simulink model "aurora_cpu_ch0_ver2_rtxsg"  (R2019b)
settings: Solver=ode45  StartTime=0.0  StopTime=1/6000  RelTol=1e-3  EnableMultiTasking=on
PreLoadFcn:
  | period=5e-9;
InitFcn:
  | period=5e-9;
undefined symbols (not defined in the file): DUALSFP, EX, opGetFPGAPeriod, VC707_2
libraries: xbsIndex_r4 x170, rtxsg_tools x22, rtxsg_communication x3, rtxsg_common x3, HighSpeedCommIO_lib x2, rtxsg_serdes_lib x2, vc707_lib x1
(part 4 of 4)

== system aurora_cpu_ch0_ver2_rtxsg/SOF_detector ==
  ready : Inport
  last : Inport  Port=2
  Inverter4 : xbsIndex_r4/Inverter  en=off  latency=0  dbl_ovrd=off  block_type=inv
  Logical1 : xbsIndex_r4/Logical  logical_function=OR  inputs=2  en=off  latency=0  precision=Full  arith_type=Unsigned  n_bits=16  bin_pt=0  align_bp=on  dbl_ovrd=off  block_type=logical
  Logical5 : xbsIndex_r4/Logical  logical_function=AND  inputs=2  en=off  latency=0  precision=Full  arith_type=Unsigned  n_bits=16  bin_pt=0  align_bp=on  dbl_ovrd=off  block_type=logical
  Register3 : xbsIndex_r4/Register  init=0  rst=on  en=off  dbl_ovrd=off  block_type=register
  startofframe : Outport
  wires:
  Register3/1 -> Logical1/1, Inverter4/1
  ready/1 -> Logical1/2, Logical5/2
  Inverter4/1 -> Logical5/1
  Logical1/1 -> Register3/1
  Logical5/1 -> startofframe/1
  last/1 -> Register3/2

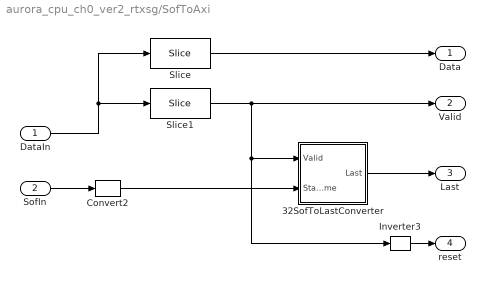
== system aurora_cpu_ch0_ver2_rtxsg/SofToAxi ==
  DataIn : Inport
  SofIn : Inport  Port=2
  32SofToLastConverter : Subsystem
  Convert2 : xbsIndex_r4/Convert  gui_display_data_type=Boolean  arith_type=Boolean  n_bits=16  bin_pt=14  float_type=Single  exp_bits=8  fraction_bits=24  quantization=Truncate  overflow=Wrap  en=off  latency=0  pipeline=off  dbl_ovrd=off  block_type=convert
  Inverter3 : xbsIndex_r4/Inverter  en=off  latency=0  dbl_ovrd=off  block_type=inv
  Slice : xbsIndex_r4/Slice  nbits=32  boolean_output=off  mode=Upper Bit Location + Width  bit1=31  base1=LSB of Input  bit0=0  base0=LSB of Input  dbl_ovrd=off  block_type=slice
  Slice1 : xbsIndex_r4/Slice  nbits=1  boolean_output=on  mode=Upper Bit Location + Width  bit1=32  base1=LSB of Input  bit0=32  base0=LSB of Input  dbl_ovrd=off  block_type=slice
  Data : Outport
  Valid : Outport  Port=2
  Last : Outport  Port=3
  reset : Outport  Port=4
  wires:
  DataIn/1 -> Slice/1, Slice1/1
  32SofToLastConverter/1(Last) -> Last/1
  Convert2/1 -> 32SofToLastConverter/2(StartOfFrame)
  Slice1/1 -> Valid/1, Inverter3/1, 32SofToLastConverter/1(Valid)
  Slice/1 -> Data/1
  SofIn/1 -> Convert2/1
  Inverter3/1 -> reset/1

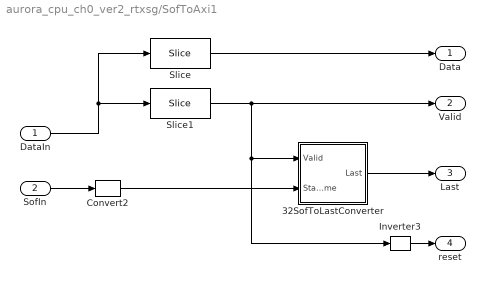
== system aurora_cpu_ch0_ver2_rtxsg/SofToAxi1 ==
  DataIn : Inport
  SofIn : Inport  Port=2
  32SofToLastConverter : Subsystem
  Convert2 : xbsIndex_r4/Convert  gui_display_data_type=Boolean  arith_type=Boolean  n_bits=16  bin_pt=14  float_type=Single  exp_bits=8  fraction_bits=24  quantization=Truncate  overflow=Wrap  en=off  latency=0  pipeline=off  dbl_ovrd=off  block_type=convert
  Inverter3 : xbsIndex_r4/Inverter  en=off  latency=0  dbl_ovrd=off  block_type=inv
  Slice : xbsIndex_r4/Slice  nbits=32  boolean_output=off  mode=Upper Bit Location + Width  bit1=31  base1=LSB of Input  bit0=0  base0=LSB of Input  dbl_ovrd=off  block_type=slice
  Slice1 : xbsIndex_r4/Slice  nbits=1  boolean_output=on  mode=Upper Bit Location + Width  bit1=32  base1=LSB of Input  bit0=32  base0=LSB of Input  dbl_ovrd=off  block_type=slice
  Data : Outport
  Valid : Outport  Port=2
  Last : Outport  Port=3
  reset : Outport  Port=4
  wires:
  DataIn/1 -> Slice/1, Slice1/1
  32SofToLastConverter/1(Last) -> Last/1
  Convert2/1 -> 32SofToLastConverter/2(StartOfFrame)
  Slice1/1 -> Valid/1, Inverter3/1, 32SofToLastConverter/1(Valid)
  Slice/1 -> Data/1
  SofIn/1 -> Convert2/1
  Inverter3/1 -> reset/1

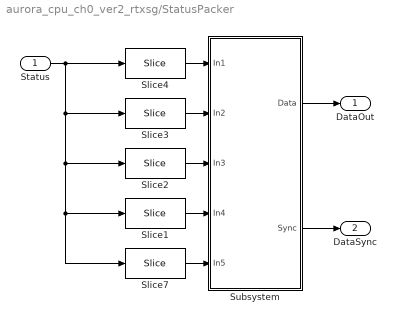
== system aurora_cpu_ch0_ver2_rtxsg/StatusPacker ==
  Status : Inport
  Slice1 : xbsIndex_r4/Slice  nbits=16  boolean_output=off  mode=Lower Bit Location + Width  bit1=0  base1=MSB of Input  bit0=80  base0=LSB of Input  dbl_ovrd=off  block_type=slice
  Slice2 : xbsIndex_r4/Slice  nbits=32  boolean_output=off  mode=Lower Bit Location + Width  bit1=0  base1=MSB of Input  bit0=48  base0=LSB of Input  dbl_ovrd=off  block_type=slice
  Slice3 : xbsIndex_r4/Slice  nbits=16  boolean_output=off  mode=Lower Bit Location + Width  bit1=0  base1=MSB of Input  bit0=32  base0=LSB of Input  dbl_ovrd=off  block_type=slice
  Slice4 : xbsIndex_r4/Slice  nbits=32  boolean_output=off  mode=Lower Bit Location + Width  bit1=0  base1=MSB of Input  bit0=0  base0=LSB of Input  dbl_ovrd=off  block_type=slice
  Slice7 : xbsIndex_r4/Slice  nbits=6  boolean_output=off  mode=Lower Bit Location + Width  bit1=0  base1=MSB of Input  bit0=96  base0=LSB of Input  dbl_ovrd=off  block_type=slice
  Subsystem : Subsystem
  DataOut : Outport
  DataSync : Outport  Port=2
  wires:
  Subsystem/1(Data) -> DataOut/1
  Subsystem/2(Sync) -> DataSync/1
  Status/1 -> Slice4/1, Slice3/1, Slice2/1, Slice1/1, Slice7/1
  Slice4/1 -> Subsystem/1(In1)
  Slice3/1 -> Subsystem/2(In2)
  Slice2/1 -> Subsystem/3(In3)
  Slice1/1 -> Subsystem/4(In4)
  Slice7/1 -> Subsystem/5(In5)

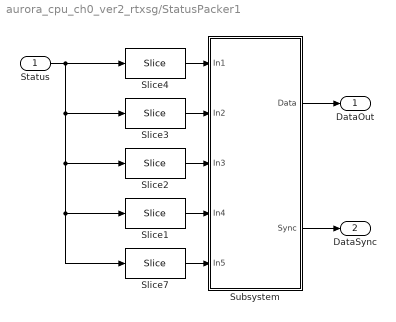
== system aurora_cpu_ch0_ver2_rtxsg/StatusPacker1 ==
  Status : Inport
  Slice1 : xbsIndex_r4/Slice  nbits=16  boolean_output=off  mode=Lower Bit Location + Width  bit1=0  base1=MSB of Input  bit0=80  base0=LSB of Input  dbl_ovrd=off  block_type=slice
  Slice2 : xbsIndex_r4/Slice  nbits=32  boolean_output=off  mode=Lower Bit Location + Width  bit1=0  base1=MSB of Input  bit0=48  base0=LSB of Input  dbl_ovrd=off  block_type=slice
  Slice3 : xbsIndex_r4/Slice  nbits=16  boolean_output=off  mode=Lower Bit Location + Width  bit1=0  base1=MSB of Input  bit0=32  base0=LSB of Input  dbl_ovrd=off  block_type=slice
  Slice4 : xbsIndex_r4/Slice  nbits=32  boolean_output=off  mode=Lower Bit Location + Width  bit1=0  base1=MSB of Input  bit0=0  base0=LSB of Input  dbl_ovrd=off  block_type=slice
  Slice7 : xbsIndex_r4/Slice  nbits=6  boolean_output=off  mode=Lower Bit Location + Width  bit1=0  base1=MSB of Input  bit0=96  base0=LSB of Input  dbl_ovrd=off  block_type=slice
  Subsystem : Subsystem
  DataOut : Outport
  DataSync : Outport  Port=2
  wires:
  Subsystem/1(Data) -> DataOut/1
  Subsystem/2(Sync) -> DataSync/1
  Status/1 -> Slice4/1, Slice3/1, Slice2/1, Slice1/1, Slice7/1
  Slice4/1 -> Subsystem/1(In1)
  Slice3/1 -> Subsystem/2(In2)
  Slice2/1 -> Subsystem/3(In3)
  Slice1/1 -> Subsystem/4(In4)
  Slice7/1 -> Subsystem/5(In5)

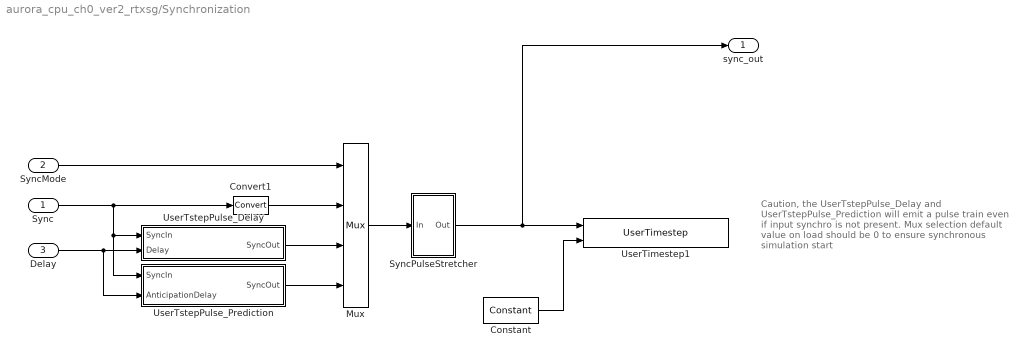
== system aurora_cpu_ch0_ver2_rtxsg/Synchronization ==
  note: Caution, the UserTstepPulse_Delay and
      | UserTstepPulse_Prediction will emit a pulse train
      | even if input synchro is not present. Mux selection
      | default value on load should be 0 to ensure
      | synchronous simulation start
  Sync : Inport
  SyncMode : Inport  Port=2
  Delay : Inport  Port=3
  Constant : xbsIndex_r4/Constant  const=1.0  gui_display_data_type=Fixed-point  arith_type=Unsigned  n_bits=1  bin_pt=0  preci_type=Single  exp_width=8  frac_width=24  explicit_period=on  period=opGetFPGAPeriod(bdroot)  equ=P=C  opselect=C  inp2=PCIN>>17  opr=+  inp1=P  carry=CIN  dbl_ovrd=off  block_type=constant
  Convert1 : xbsIndex_r4/Convert  gui_display_data_type=Boolean  arith_type=Boolean  n_bits=1  bin_pt=0  float_type=Single  exp_bits=8  fraction_bits=24  quantization=Truncate  overflow=Wrap  en=off  latency=0  pipeline=off  dbl_ovrd=off  block_type=convert
  Mux : xbsIndex_r4/Mux  inputs=3  en=off  latency=0  precision=Full  arith_type=Unsigned  n_bits=16  bin_pt=14  quantization=Truncate  overflow=Wrap  dbl_ovrd=off  block_type=mux
  SyncPulseStretcher : Subsystem
  UserTimestep1 : vc707_lib/UserTimestep  SyncSelControl=From Input Port  SamplePeriod=opGetFPGAPeriod(bdroot)
      link override SyncSelCtrl: const=0  gui_display_data_type=Fixed-point  arith_type=Unsigned  n_bits=1  bin_pt=0  preci_type=Single  exp_width=8  frac_width=24  explicit_period=on  period=SamplePeriod  equ=P=C  opselect=C  inp2=PCIN>>17  opr=+  inp1=P  carry=CIN  dbl_ovrd=off
      settings: SourceProductName=RT-XSG
  UserTstepPulse_Delay : Subsystem
  UserTstepPulse_Prediction : Subsystem
  sync_out : Outport
  wires:
  Sync/1 -> UserTstepPulse_Prediction/1(SyncIn), UserTstepPulse_Delay/1(SyncIn), Convert1/1
  SyncMode/1 -> Mux/1
  Delay/1 -> UserTstepPulse_Prediction/2(AnticipationDelay), UserTstepPulse_Delay/2(Delay)
  Convert1/1 -> Mux/2
  UserTstepPulse_Delay/1(SyncOut) -> Mux/3
  UserTstepPulse_Prediction/1(SyncOut) -> Mux/4
  SyncPulseStretcher/1(Out) -> sync_out/1, UserTimestep1/1
  Constant/1 -> UserTimestep1/2
  Mux/1 -> SyncPulseStretcher/1(In)

== system aurora_cpu_ch0_ver2_rtxsg/TimeStepSwitch ==
  MasterTimeStep : Inport
  InitTimeStep : Inport  Port=2
  Logical : xbsIndex_r4/Logical  logical_function=OR  inputs=2  en=off  latency=0  precision=Full  arith_type=Unsigned  n_bits=16  bin_pt=0  align_bp=on  dbl_ovrd=off  block_type=logical
  Mux : xbsIndex_r4/Mux  inputs=2  en=off  latency=0  precision=Full  arith_type=Unsigned  n_bits=16  bin_pt=14  quantization=Truncate  overflow=Wrap  dbl_ovrd=off  block_type=mux
  Register : xbsIndex_r4/Register  init=0  rst=off  en=off  dbl_ovrd=off  block_type=register
  TimeStep : Outport
  wires:
  Register/1 -> Logical/1
  MasterTimeStep/1 -> Logical/2, Mux/3
  Logical/1 -> Mux/1, Register/1
  Mux/1 -> TimeStep/1
  InitTimeStep/1 -> Mux/2

== system aurora_cpu_ch0_ver2_rtxsg/TimestepGenerator ==
  Constant3 : xbsIndex_r4/Constant  const=5000  gui_display_data_type=Fixed-point  arith_type=Unsigned  n_bits=32  bin_pt=0  preci_type=Single  exp_width=8  frac_width=24  explicit_period=on  period=opGetFPGAPeriod(bdroot)  equ=P=C  opselect=C  inp2=PCIN>>17  opr=+  inp1=P  carry=CIN  dbl_ovrd=off  block_type=constant
  Counter1 : xbsIndex_r4/Counter  cnt_type=Free Running  cnt_to=50e-6/1e-9  operation=Up  start_count=0  cnt_by_val=1  arith_type=Unsigned  n_bits=32  bin_pt=0  load_pin=off  rst=on  en=off  explicit_period=on  period=opGetFPGAPeriod(bdroot)  use_behavioral_HDL=off  implementation=Fabric  dbl_ovrd=off  block_type=counter
  Relational : xbsIndex_r4/Relational  mode=a=b  op_type=Bool  en=off  latency=0  dbl_ovrd=off  block_type=relational
  TimeStep : Outport
  wires:
  Relational/1 -> TimeStep/1, Counter1/1
  Constant3/1 -> Relational/2
  Counter1/1 -> Relational/1

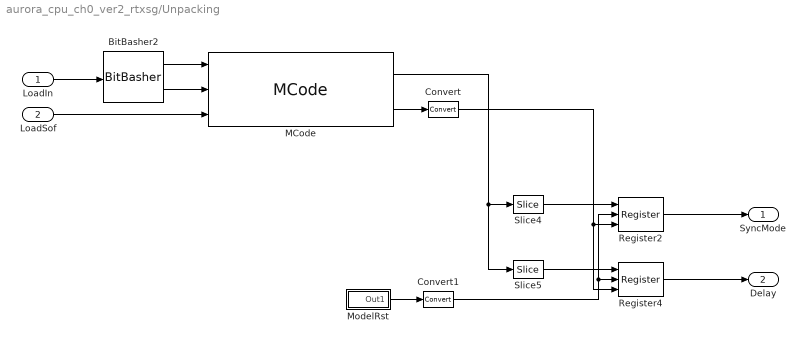
== system aurora_cpu_ch0_ver2_rtxsg/Unpacking ==
  LoadIn : Inport
  LoadSof : Inport  Port=2
  BitBasher2 : xbsIndex_r4/BitBasher  bitexpr=|  display_expr=off  sr_1=1  arith_type1=Unsigned  bin_pt1=0  sr_2=2  arith_type2=Unsigned  bin_pt2=0  sr_3=3  arith_type3=Unsigned  bin_pt3=0  sr_4=4  arith_type4=Unsigned  bin_pt4=0  dbl_ovrd=off  block_type=bitbasher
      | <!DOCTYPE HTML PUBLIC "-//W3C//DTD HTML 4.0//EN" "http://www.w3.org/TR/REC-html40/strict.dtd">
      | <html><head><meta name="qrichtext" content="1" /><style type="text/css">
      | p, li { white-space: pre-wrap; }
      | </style></head><body style=" font-family:'MS Shell Dlg 2'; font-size:8.25pt; font-weight:400; font-style:normal;">
      | <p style=" margin-top:12px; margin-bottom:12px; margin-left:0px; margin-right:0px; -qt-block-indent:0; text-indent:0px;"><span style=" font-family:'MS Shell Dlg'; font-size:8pt;">data={i[31:0]}<br />valid={i[32]}</span></p></body></html>
  Convert : xbsIndex_r4/Convert  gui_display_data_type=Boolean  arith_type=Boolean  n_bits=16  bin_pt=14  float_type=Single  exp_bits=8  fraction_bits=24  quantization=Truncate  overflow=Wrap  en=off  latency=0  pipeline=off  dbl_ovrd=off  block_type=convert
  Convert1 : xbsIndex_r4/Convert  gui_display_data_type=Boolean  arith_type=Boolean  n_bits=16  bin_pt=14  float_type=Single  exp_bits=8  fraction_bits=24  quantization=Truncate  overflow=Wrap  en=off  latency=0  pipeline=off  dbl_ovrd=off  block_type=convert
  MCode : xbsIndex_r4/MCode  mfname=efsUnpackingDesequencerSof  explicit_period=off  period=1  inputsTable={'boundInpExpr'=>['2','','',''],'inputs'=>['NbElements','Output_in','WE','Sof']}  outputsTable={'outputs'=>['Output_cat','OutputUpdated'],'suppressOut'=>['off','off']}  enable_stdout=off  enable_debug=off  suppress_output=on  defparams={'NbElements',2}  hide_port_list={}  dbl_ovrd=off  block_type=mcode
  ModelRst : Subsystem
  Register2 : xbsIndex_r4/Register  init=0  rst=on  en=on  dbl_ovrd=off  block_type=register
  Register4 : xbsIndex_r4/Register  init=0  rst=on  en=on  dbl_ovrd=off  block_type=register
  Slice4 : xbsIndex_r4/Slice  nbits=2  boolean_output=off  mode=Lower Bit Location + Width  bit1=0  base1=MSB of Input  bit0=0  base0=LSB of Input  dbl_ovrd=off  block_type=slice
  Slice5 : xbsIndex_r4/Slice  nbits=22  boolean_output=off  mode=Lower Bit Location + Width  bit1=0  base1=MSB of Input  bit0=2  base0=LSB of Input  dbl_ovrd=off  block_type=slice
  SyncMode : Outport
  Delay : Outport  Port=2
  wires:
  BitBasher2/1 -> MCode/1
  BitBasher2/2 -> MCode/2
  LoadIn/1 -> BitBasher2/1
  LoadSof/1 -> MCode/3
  ModelRst/1(Out1) -> Convert1/1
  MCode/2 -> Convert/1
  MCode/1 -> Slice4/1, Slice5/1
  Register2/1 -> SyncMode/1
  Register4/1 -> Delay/1
  Slice4/1 -> Register2/1
  Slice5/1 -> Register4/1
  Convert/1 -> Register2/3, Register4/3
  Convert1/1 -> Register2/2, Register4/2

== system aurora_cpu_ch0_ver2_rtxsg/SofToAxi/32SofToLastConverter ==
  Valid : Inport
  StartOfFrame : Inport  Port=2
  Constant2 : xbsIndex_r4/Constant  const=31  gui_display_data_type=Fixed-point  arith_type=Signed (2's comp)  n_bits=8  bin_pt=0  preci_type=Single  exp_width=8  frac_width=24  explicit_period=off  period=1  equ=P=C  opselect=C  inp2=PCIN>>17  opr=+  inp1=P  carry=CIN  dbl_ovrd=off  block_type=constant
  Counter : xbsIndex_r4/Counter  cnt_type=Free Running  cnt_to=31  operation=Up  start_count=0  cnt_by_val=1  arith_type=Unsigned  n_bits=8  bin_pt=0  load_pin=off  rst=on  en=on  explicit_period=off  period=1  use_behavioral_HDL=off  implementation=Fabric  dbl_ovrd=off  block_type=counter
  Relational1 : xbsIndex_r4/Relational  mode=a=b  op_type=Bool  en=off  latency=0  dbl_ovrd=off  block_type=relational
  Last : Outport
  wires:
  Counter/1 -> Relational1/2
  Constant2/1 -> Relational1/1
  Valid/1 -> Counter/2
  Relational1/1 -> Last/1
  StartOfFrame/1 -> Counter/1

== system aurora_cpu_ch0_ver2_rtxsg/SofToAxi1/32SofToLastConverter ==
  Valid : Inport
  StartOfFrame : Inport  Port=2
  Constant2 : xbsIndex_r4/Constant  const=31  gui_display_data_type=Fixed-point  arith_type=Signed (2's comp)  n_bits=8  bin_pt=0  preci_type=Single  exp_width=8  frac_width=24  explicit_period=off  period=1  equ=P=C  opselect=C  inp2=PCIN>>17  opr=+  inp1=P  carry=CIN  dbl_ovrd=off  block_type=constant
  Counter : xbsIndex_r4/Counter  cnt_type=Free Running  cnt_to=31  operation=Up  start_count=0  cnt_by_val=1  arith_type=Unsigned  n_bits=8  bin_pt=0  load_pin=off  rst=on  en=on  explicit_period=off  period=1  use_behavioral_HDL=off  implementation=Fabric  dbl_ovrd=off  block_type=counter
  Relational1 : xbsIndex_r4/Relational  mode=a=b  op_type=Bool  en=off  latency=0  dbl_ovrd=off  block_type=relational
  Last : Outport
  wires:
  Counter/1 -> Relational1/2
  Constant2/1 -> Relational1/1
  Valid/1 -> Counter/2
  Relational1/1 -> Last/1
  StartOfFrame/1 -> Counter/1

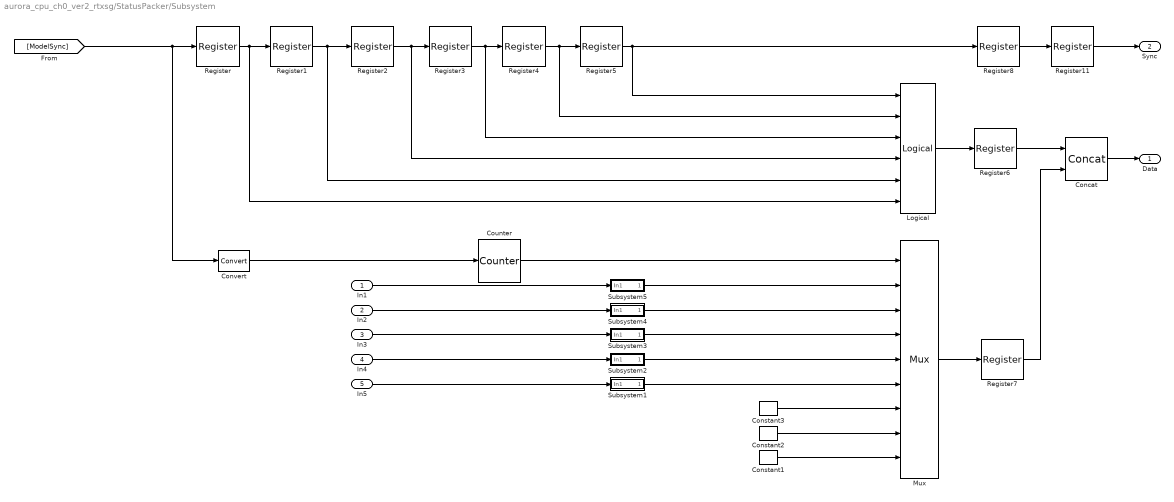
== system aurora_cpu_ch0_ver2_rtxsg/StatusPacker/Subsystem ==
  In1 : Inport
  In2 : Inport  Port=2
  In3 : Inport  Port=3
  In4 : Inport  Port=4
  In5 : Inport  Port=5
  Concat : xbsIndex_r4/Concat  num_inputs=2  dbl_ovrd=off  block_type=concat
  Constant1 : xbsIndex_r4/Constant  const=0  gui_display_data_type=Fixed-point  arith_type=Unsigned  n_bits=32  bin_pt=0  preci_type=Single  exp_width=8  frac_width=24  explicit_period=on  period=opGetFPGAPeriod(bdroot)  equ=P=C  opselect=C  inp2=PCIN>>17  opr=+  inp1=P  carry=CIN  dbl_ovrd=off  block_type=constant
  Constant2 : xbsIndex_r4/Constant  const=0  gui_display_data_type=Fixed-point  arith_type=Unsigned  n_bits=32  bin_pt=0  preci_type=Single  exp_width=8  frac_width=24  explicit_period=on  period=opGetFPGAPeriod(bdroot)  equ=P=C  opselect=C  inp2=PCIN>>17  opr=+  inp1=P  carry=CIN  dbl_ovrd=off  block_type=constant
  Constant3 : xbsIndex_r4/Constant  const=0  gui_display_data_type=Fixed-point  arith_type=Unsigned  n_bits=32  bin_pt=0  preci_type=Single  exp_width=8  frac_width=24  explicit_period=on  period=opGetFPGAPeriod(bdroot)  equ=P=C  opselect=C  inp2=PCIN>>17  opr=+  inp1=P  carry=CIN  dbl_ovrd=off  block_type=constant
  Convert : xbsIndex_r4/Convert  gui_display_data_type=Boolean  arith_type=Boolean  n_bits=16  bin_pt=14  float_type=Single  exp_bits=8  fraction_bits=24  quantization=Truncate  overflow=Wrap  en=off  latency=0  pipeline=off  dbl_ovrd=off  block_type=convert
  Counter : xbsIndex_r4/Counter  cnt_type=Free Running  cnt_to=Inf  operation=Up  start_count=0  cnt_by_val=1  arith_type=Unsigned  n_bits=3  bin_pt=0  load_pin=off  rst=on  en=off  explicit_period=on  period=opGetFPGAPeriod(bdroot)  use_behavioral_HDL=off  implementation=Fabric  dbl_ovrd=off  block_type=counter
  Logical : xbsIndex_r4/Logical  logical_function=OR  inputs=6  en=off  latency=0  precision=Full  arith_type=Unsigned  n_bits=16  bin_pt=0  align_bp=on  dbl_ovrd=off  block_type=logical
  Mux : xbsIndex_r4/Mux  inputs=8  en=off  latency=0  precision=Full  arith_type=Unsigned  n_bits=16  bin_pt=14  quantization=Truncate  overflow=Wrap  dbl_ovrd=off  block_type=mux
  Register{,1..8,11} (10 alike) : xbsIndex_r4/Register  init=0  rst=off  en=off  dbl_ovrd=off  block_type=register
  Subsystem1 : Subsystem
  Subsystem2 : Subsystem
  Subsystem3 : Subsystem
  Subsystem4 : Subsystem
  Subsystem5 : Subsystem
  Data : Outport
  Sync : Outport  Port=2
  wires:
  Convert/1 -> Counter/1
  Concat/1 -> Data/1
  Register7/1 -> Concat/2
  Register6/1 -> Concat/1
  Counter/1 -> Mux/1
  In5/1 -> Subsystem1/1(In1)
  In4/1 -> Subsystem2/1(In1)
  In3/1 -> Subsystem3/1(In1)
  In2/1 -> Subsystem4/1(In1)
  In1/1 -> Subsystem5/1(In1)
  Mux/1 -> Register7/1
  Logical/1 -> Register6/1
  [ModelSync] -> Convert/1, Register/1
  Register5/1 -> Register8/1, Logical/1
  Register4/1 -> Register5/1, Logical/2
  Register3/1 -> Register4/1, Logical/3
  Register2/1 -> Register3/1, Logical/4
  Register1/1 -> Register2/1, Logical/5
  Register/1 -> Register1/1, Logical/6
  Register8/1 -> Register11/1
  Register11/1 -> Sync/1
  Constant2/1 -> Mux/8
  Constant1/1 -> Mux/9
  Subsystem1/1(Out1) -> Mux/6
  Subsystem2/1(Out1) -> Mux/5
  Subsystem3/1(Out1) -> Mux/4
  Subsystem4/1(Out1) -> Mux/3
  Subsystem5/1(Out1) -> Mux/2
  Constant3/1 -> Mux/7

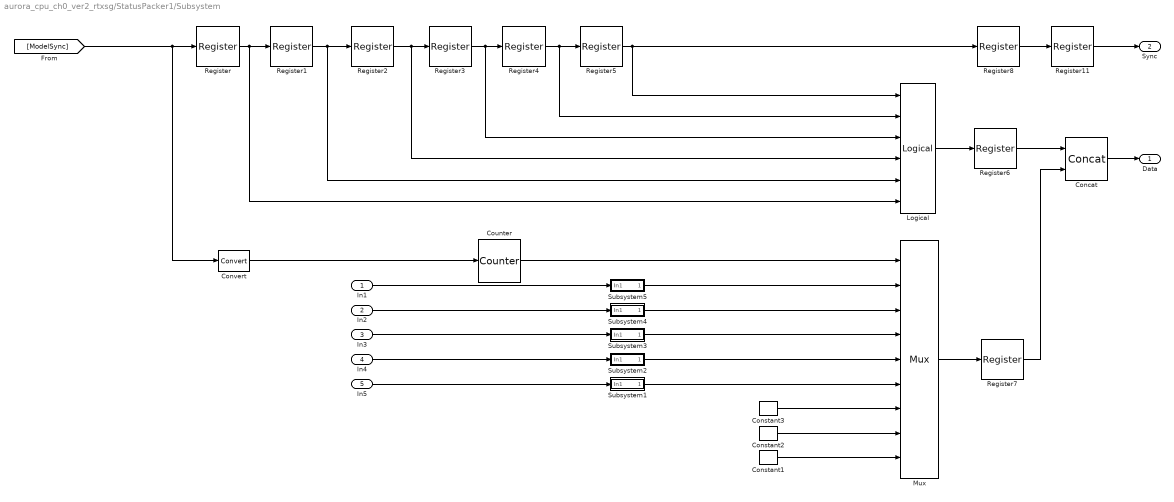
== system aurora_cpu_ch0_ver2_rtxsg/StatusPacker1/Subsystem ==
  In1 : Inport
  In2 : Inport  Port=2
  In3 : Inport  Port=3
  In4 : Inport  Port=4
  In5 : Inport  Port=5
  Concat : xbsIndex_r4/Concat  num_inputs=2  dbl_ovrd=off  block_type=concat
  Constant1 : xbsIndex_r4/Constant  const=0  gui_display_data_type=Fixed-point  arith_type=Unsigned  n_bits=32  bin_pt=0  preci_type=Single  exp_width=8  frac_width=24  explicit_period=on  period=opGetFPGAPeriod(bdroot)  equ=P=C  opselect=C  inp2=PCIN>>17  opr=+  inp1=P  carry=CIN  dbl_ovrd=off  block_type=constant
  Constant2 : xbsIndex_r4/Constant  const=0  gui_display_data_type=Fixed-point  arith_type=Unsigned  n_bits=32  bin_pt=0  preci_type=Single  exp_width=8  frac_width=24  explicit_period=on  period=opGetFPGAPeriod(bdroot)  equ=P=C  opselect=C  inp2=PCIN>>17  opr=+  inp1=P  carry=CIN  dbl_ovrd=off  block_type=constant
  Constant3 : xbsIndex_r4/Constant  const=0  gui_display_data_type=Fixed-point  arith_type=Unsigned  n_bits=32  bin_pt=0  preci_type=Single  exp_width=8  frac_width=24  explicit_period=on  period=opGetFPGAPeriod(bdroot)  equ=P=C  opselect=C  inp2=PCIN>>17  opr=+  inp1=P  carry=CIN  dbl_ovrd=off  block_type=constant
  Convert : xbsIndex_r4/Convert  gui_display_data_type=Boolean  arith_type=Boolean  n_bits=16  bin_pt=14  float_type=Single  exp_bits=8  fraction_bits=24  quantization=Truncate  overflow=Wrap  en=off  latency=0  pipeline=off  dbl_ovrd=off  block_type=convert
  Counter : xbsIndex_r4/Counter  cnt_type=Free Running  cnt_to=Inf  operation=Up  start_count=0  cnt_by_val=1  arith_type=Unsigned  n_bits=3  bin_pt=0  load_pin=off  rst=on  en=off  explicit_period=on  period=opGetFPGAPeriod(bdroot)  use_behavioral_HDL=off  implementation=Fabric  dbl_ovrd=off  block_type=counter
  Logical : xbsIndex_r4/Logical  logical_function=OR  inputs=6  en=off  latency=0  precision=Full  arith_type=Unsigned  n_bits=16  bin_pt=0  align_bp=on  dbl_ovrd=off  block_type=logical
  Mux : xbsIndex_r4/Mux  inputs=8  en=off  latency=0  precision=Full  arith_type=Unsigned  n_bits=16  bin_pt=14  quantization=Truncate  overflow=Wrap  dbl_ovrd=off  block_type=mux
  Register{,1..8,11} (10 alike) : xbsIndex_r4/Register  init=0  rst=off  en=off  dbl_ovrd=off  block_type=register
  Subsystem1 : Subsystem
  Subsystem2 : Subsystem
  Subsystem3 : Subsystem
  Subsystem4 : Subsystem
  Subsystem5 : Subsystem
  Data : Outport
  Sync : Outport  Port=2
  wires:
  Convert/1 -> Counter/1
  Concat/1 -> Data/1
  Register7/1 -> Concat/2
  Register6/1 -> Concat/1
  Counter/1 -> Mux/1
  In5/1 -> Subsystem1/1(In1)
  In4/1 -> Subsystem2/1(In1)
  In3/1 -> Subsystem3/1(In1)
  In2/1 -> Subsystem4/1(In1)
  In1/1 -> Subsystem5/1(In1)
  Mux/1 -> Register7/1
  Logical/1 -> Register6/1
  [ModelSync] -> Convert/1, Register/1
  Register5/1 -> Register8/1, Logical/1
  Register4/1 -> Register5/1, Logical/2
  Register3/1 -> Register4/1, Logical/3
  Register2/1 -> Register3/1, Logical/4
  Register1/1 -> Register2/1, Logical/5
  Register/1 -> Register1/1, Logical/6
  Register8/1 -> Register11/1
  Register11/1 -> Sync/1
  Constant2/1 -> Mux/8
  Constant1/1 -> Mux/9
  Subsystem1/1(Out1) -> Mux/6
  Subsystem2/1(Out1) -> Mux/5
  Subsystem3/1(Out1) -> Mux/4
  Subsystem4/1(Out1) -> Mux/3
  Subsystem5/1(Out1) -> Mux/2
  Constant3/1 -> Mux/7

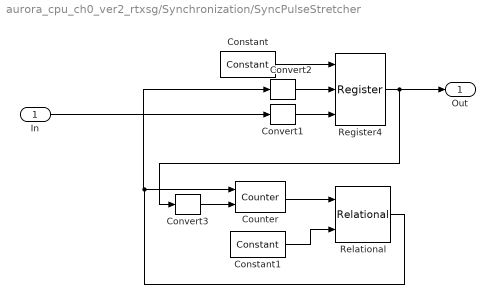
== system aurora_cpu_ch0_ver2_rtxsg/Synchronization/SyncPulseStretcher ==
  In : Inport
  Constant : xbsIndex_r4/Constant  const=1.0  gui_display_data_type=Fixed-point  arith_type=Unsigned  n_bits=1  bin_pt=0  preci_type=Single  exp_width=8  frac_width=24  explicit_period=on  period=opGetFPGAPeriod(bdroot)  equ=P=C  opselect=C  inp2=PCIN>>17  opr=+  inp1=P  carry=CIN  dbl_ovrd=off  block_type=constant
  Constant1 : xbsIndex_r4/Constant  const=13  gui_display_data_type=Fixed-point  arith_type=Unsigned  n_bits=4  bin_pt=0  preci_type=Single  exp_width=8  frac_width=24  explicit_period=on  period=opGetFPGAPeriod(bdroot)  equ=P=C  opselect=C  inp2=PCIN>>17  opr=+  inp1=P  carry=CIN  dbl_ovrd=off  block_type=constant
  Convert1 : xbsIndex_r4/Convert  gui_display_data_type=Boolean  arith_type=Boolean  n_bits=16  bin_pt=14  float_type=Single  exp_bits=8  fraction_bits=24  quantization=Truncate  overflow=Wrap  en=off  latency=0  pipeline=off  dbl_ovrd=off  block_type=convert
  Convert2 : xbsIndex_r4/Convert  gui_display_data_type=Boolean  arith_type=Boolean  n_bits=16  bin_pt=14  float_type=Single  exp_bits=8  fraction_bits=24  quantization=Truncate  overflow=Wrap  en=off  latency=0  pipeline=off  dbl_ovrd=off  block_type=convert
  Convert3 : xbsIndex_r4/Convert  gui_display_data_type=Boolean  arith_type=Boolean  n_bits=16  bin_pt=14  float_type=Single  exp_bits=8  fraction_bits=24  quantization=Truncate  overflow=Wrap  en=off  latency=0  pipeline=off  dbl_ovrd=off  block_type=convert
  Counter : xbsIndex_r4/Counter  cnt_type=Free Running  cnt_to=Inf  operation=Up  start_count=0  cnt_by_val=1  arith_type=Unsigned  n_bits=4  bin_pt=0  load_pin=off  rst=on  en=on  explicit_period=on  period=opGetFPGAPeriod(bdroot)  use_behavioral_HDL=off  implementation=Fabric  dbl_ovrd=off  block_type=counter
  Register4 : xbsIndex_r4/Register  init=0  rst=on  en=on  dbl_ovrd=off  block_type=register
  Relational : xbsIndex_r4/Relational  mode=a>b  op_type=Bool  en=off  latency=1  dbl_ovrd=off  block_type=relational
  Out : Outport
  wires:
  In/1 -> Convert1/1
  Constant/1 -> Register4/1
  Counter/1 -> Relational/1
  Constant1/1 -> Relational/2
  Relational/1 -> Convert2/1, Counter/1
  Register4/1 -> Convert3/1, Out/1
  Convert3/1 -> Counter/2
  Convert2/1 -> Register4/2
  Convert1/1 -> Register4/3

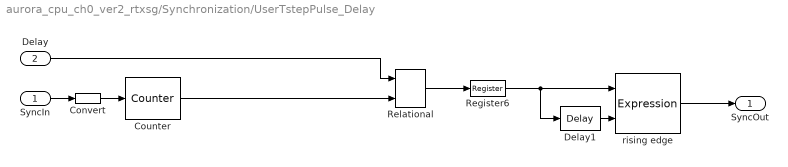
== system aurora_cpu_ch0_ver2_rtxsg/Synchronization/UserTstepPulse_Delay ==
  SyncIn : Inport
  Delay : Inport  Port=2
  Convert : xbsIndex_r4/Convert  gui_display_data_type=Boolean  arith_type=Boolean  n_bits=16  bin_pt=14  float_type=Single  exp_bits=8  fraction_bits=24  quantization=Truncate  overflow=Wrap  en=off  latency=0  pipeline=off  dbl_ovrd=off  block_type=convert
  Counter : xbsIndex_r4/Counter  cnt_type=Count Limited  cnt_to=2^22-1  operation=Up  start_count=0  cnt_by_val=1  arith_type=Unsigned  n_bits=22  bin_pt=0  load_pin=off  rst=on  en=off  explicit_period=on  period=opGetFPGAPeriod(bdroot)  use_behavioral_HDL=off  implementation=Fabric  dbl_ovrd=off  block_type=counter
  Delay1 : xbsIndex_r4/Delay  rst=off  infoeditControl=Selection of Reset will increase slice count due to use of real FFs and instead of SRLs  en=off  latency=1  reg_retiming=off  dbl_ovrd=off  block_type=delay
  Register6 : xbsIndex_r4/Register  init=0  rst=off  en=off  dbl_ovrd=off  block_type=register
  Relational : xbsIndex_r4/Relational  mode=a=b  op_type=Bool  en=off  latency=0  dbl_ovrd=off  block_type=relational
  rising edge : xbsIndex_r4/Expression  expression=a & ~b  align_bp=on  en=off  latency=0  precision=Full  arith_type=Unsigned  n_bits=16  bin_pt=0  dbl_ovrd=off  block_type=expr
  SyncOut : Outport
  wires:
  Register6/1 -> rising edge/1, Delay1/1
  rising edge/1 -> SyncOut/1
  Delay1/1 -> rising edge/2
  SyncIn/1 -> Convert/1
  Convert/1 -> Counter/1
  Counter/1 -> Relational/2
  Delay/1 -> Relational/1
  Relational/1 -> Register6/1

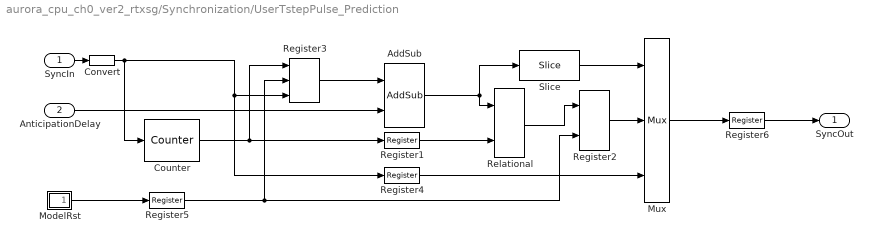
== system aurora_cpu_ch0_ver2_rtxsg/Synchronization/UserTstepPulse_Prediction ==
  SyncIn : Inport
  AnticipationDelay : Inport  Port=2
  AddSub : xbsIndex_r4/AddSub  mode=Subtraction  use_carryin=off  use_carryout=off  en=off  latency=1  precision=Full  arith_type=Unsigned  n_bits=16  bin_pt=14  quantization=Truncate  overflow=Wrap  use_behavioral_HDL=off  hw_selection=Fabric  pipelined=off  dbl_ovrd=off  block_type=addsub
  Convert : xbsIndex_r4/Convert  gui_display_data_type=Boolean  arith_type=Boolean  n_bits=16  bin_pt=14  float_type=Single  exp_bits=8  fraction_bits=24  quantization=Truncate  overflow=Wrap  en=off  latency=0  pipeline=off  dbl_ovrd=off  block_type=convert
  Counter : xbsIndex_r4/Counter  cnt_type=Count Limited  cnt_to=2^22-1  operation=Up  start_count=0  cnt_by_val=1  arith_type=Unsigned  n_bits=22  bin_pt=0  load_pin=off  rst=on  en=off  explicit_period=on  period=opGetFPGAPeriod(bdroot)  use_behavioral_HDL=off  implementation=Fabric  dbl_ovrd=off  block_type=counter
  ModelRst : Subsystem
  Mux : xbsIndex_r4/Mux  inputs=2  en=off  latency=0  precision=Full  arith_type=Unsigned  n_bits=16  bin_pt=14  quantization=Truncate  overflow=Wrap  dbl_ovrd=off  block_type=mux
  Register{1,4..6} (4 alike) : xbsIndex_r4/Register  init=0  rst=off  en=off  dbl_ovrd=off  block_type=register
  Register2 : xbsIndex_r4/Register  init=0  rst=on  en=off  dbl_ovrd=off  block_type=register
  Register3 : xbsIndex_r4/Register  init=0  rst=on  en=on  dbl_ovrd=off  block_type=register
  Relational : xbsIndex_r4/Relational  mode=a=b  op_type=Bool  en=off  latency=0  dbl_ovrd=off  block_type=relational
  Slice : xbsIndex_r4/Slice  nbits=1  boolean_output=off  mode=Upper Bit Location + Width  bit1=0  base1=MSB of Input  bit0=0  base0=LSB of Input  dbl_ovrd=off  block_type=slice
  SyncOut : Outport
  wires:
  Register6/1 -> SyncOut/1
  Mux/1 -> Register6/1
  Register5/1 -> Register3/2, Register2/2
  ModelRst/1(Rst) -> Register5/1
  Slice/1 -> Mux/1
  Register4/1 -> Mux/3
  Register2/1 -> Mux/2
  Relational/1 -> Register2/1
  AddSub/1 -> Slice/1, Relational/1
  AnticipationDelay/1 -> AddSub/2
  Register1/1 -> Relational/2
  Counter/1 -> Register1/1, Register3/1
  Register3/1 -> AddSub/1
  Convert/1 -> Register3/3, Register4/1, Counter/1
  SyncIn/1 -> Convert/1

== system aurora_cpu_ch0_ver2_rtxsg/Unpacking/ModelRst ==
  Simulation State : rtxsg_common/Simulation State  TimerWidth=22
      settings: SourceProductName=RT-XSG
  Terminator{,1..4} (5 alike) : Terminator
  Out1 : Outport
  wires:
  Simulation State/1 -> Terminator/1
  Simulation State/2 -> Terminator1/1
  Simulation State/3 -> Terminator2/1
  Simulation State/5 -> Terminator3/1
  Simulation State/6 -> Terminator4/1
  Simulation State/4 -> Out1/1

== system aurora_cpu_ch0_ver2_rtxsg/StatusPacker/Subsystem/Subsystem1 ==
  In1 : Inport
  Concat1 : xbsIndex_r4/Concat  num_inputs=2  dbl_ovrd=off  block_type=concat
  Constant3 : xbsIndex_r4/Constant  const=0  gui_display_data_type=Fixed-point  arith_type=Unsigned  n_bits=32  bin_pt=0  preci_type=Single  exp_width=8  frac_width=24  explicit_period=on  period=opGetFPGAPeriod(bdroot)  equ=P=C  opselect=C  inp2=PCIN>>17  opr=+  inp1=P  carry=CIN  dbl_ovrd=off  block_type=constant
  Slice : xbsIndex_r4/Slice  nbits=32  boolean_output=off  mode=Lower Bit Location + Width  bit1=0  base1=MSB of Input  bit0=0  base0=LSB of Input  dbl_ovrd=off  block_type=slice
  Out1 : Outport
  wires:
  In1/1 -> Concat1/2
  Slice/1 -> Out1/1
  Constant3/1 -> Concat1/1
  Concat1/1 -> Slice/1

== system aurora_cpu_ch0_ver2_rtxsg/StatusPacker/Subsystem/Subsystem2 ==
  In1 : Inport
  Concat1 : xbsIndex_r4/Concat  num_inputs=2  dbl_ovrd=off  block_type=concat
  Constant3 : xbsIndex_r4/Constant  const=0  gui_display_data_type=Fixed-point  arith_type=Unsigned  n_bits=32  bin_pt=0  preci_type=Single  exp_width=8  frac_width=24  explicit_period=on  period=opGetFPGAPeriod(bdroot)  equ=P=C  opselect=C  inp2=PCIN>>17  opr=+  inp1=P  carry=CIN  dbl_ovrd=off  block_type=constant
  Slice : xbsIndex_r4/Slice  nbits=32  boolean_output=off  mode=Lower Bit Location + Width  bit1=0  base1=MSB of Input  bit0=0  base0=LSB of Input  dbl_ovrd=off  block_type=slice
  Out1 : Outport
  wires:
  Concat1/1 -> Slice/1
  Constant3/1 -> Concat1/1
  Slice/1 -> Out1/1
  In1/1 -> Concat1/2

== system aurora_cpu_ch0_ver2_rtxsg/StatusPacker/Subsystem/Subsystem3 ==
  In1 : Inport
  Concat1 : xbsIndex_r4/Concat  num_inputs=2  dbl_ovrd=off  block_type=concat
  Constant3 : xbsIndex_r4/Constant  const=0  gui_display_data_type=Fixed-point  arith_type=Unsigned  n_bits=32  bin_pt=0  preci_type=Single  exp_width=8  frac_width=24  explicit_period=on  period=opGetFPGAPeriod(bdroot)  equ=P=C  opselect=C  inp2=PCIN>>17  opr=+  inp1=P  carry=CIN  dbl_ovrd=off  block_type=constant
  Slice : xbsIndex_r4/Slice  nbits=32  boolean_output=off  mode=Lower Bit Location + Width  bit1=0  base1=MSB of Input  bit0=0  base0=LSB of Input  dbl_ovrd=off  block_type=slice
  Out1 : Outport
  wires:
  In1/1 -> Concat1/2
  Slice/1 -> Out1/1
  Constant3/1 -> Concat1/1
  Concat1/1 -> Slice/1

== system aurora_cpu_ch0_ver2_rtxsg/StatusPacker/Subsystem/Subsystem4 ==
  In1 : Inport
  Concat1 : xbsIndex_r4/Concat  num_inputs=2  dbl_ovrd=off  block_type=concat
  Constant3 : xbsIndex_r4/Constant  const=0  gui_display_data_type=Fixed-point  arith_type=Unsigned  n_bits=32  bin_pt=0  preci_type=Single  exp_width=8  frac_width=24  explicit_period=on  period=opGetFPGAPeriod(bdroot)  equ=P=C  opselect=C  inp2=PCIN>>17  opr=+  inp1=P  carry=CIN  dbl_ovrd=off  block_type=constant
  Slice : xbsIndex_r4/Slice  nbits=32  boolean_output=off  mode=Lower Bit Location + Width  bit1=0  base1=MSB of Input  bit0=0  base0=LSB of Input  dbl_ovrd=off  block_type=slice
  Out1 : Outport
  wires:
  Concat1/1 -> Slice/1
  Constant3/1 -> Concat1/1
  Slice/1 -> Out1/1
  In1/1 -> Concat1/2

== system aurora_cpu_ch0_ver2_rtxsg/StatusPacker/Subsystem/Subsystem5 ==
  In1 : Inport
  Concat1 : xbsIndex_r4/Concat  num_inputs=2  dbl_ovrd=off  block_type=concat
  Constant3 : xbsIndex_r4/Constant  const=0  gui_display_data_type=Fixed-point  arith_type=Unsigned  n_bits=32  bin_pt=0  preci_type=Single  exp_width=8  frac_width=24  explicit_period=on  period=opGetFPGAPeriod(bdroot)  equ=P=C  opselect=C  inp2=PCIN>>17  opr=+  inp1=P  carry=CIN  dbl_ovrd=off  block_type=constant
  Slice : xbsIndex_r4/Slice  nbits=32  boolean_output=off  mode=Lower Bit Location + Width  bit1=0  base1=MSB of Input  bit0=0  base0=LSB of Input  dbl_ovrd=off  block_type=slice
  Out1 : Outport
  wires:
  In1/1 -> Concat1/2
  Slice/1 -> Out1/1
  Constant3/1 -> Concat1/1
  Concat1/1 -> Slice/1

== system aurora_cpu_ch0_ver2_rtxsg/StatusPacker1/Subsystem/Subsystem1 ==
  In1 : Inport
  Concat1 : xbsIndex_r4/Concat  num_inputs=2  dbl_ovrd=off  block_type=concat
  Constant3 : xbsIndex_r4/Constant  const=0  gui_display_data_type=Fixed-point  arith_type=Unsigned  n_bits=32  bin_pt=0  preci_type=Single  exp_width=8  frac_width=24  explicit_period=on  period=opGetFPGAPeriod(bdroot)  equ=P=C  opselect=C  inp2=PCIN>>17  opr=+  inp1=P  carry=CIN  dbl_ovrd=off  block_type=constant
  Slice : xbsIndex_r4/Slice  nbits=32  boolean_output=off  mode=Lower Bit Location + Width  bit1=0  base1=MSB of Input  bit0=0  base0=LSB of Input  dbl_ovrd=off  block_type=slice
  Out1 : Outport
  wires:
  In1/1 -> Concat1/2
  Slice/1 -> Out1/1
  Constant3/1 -> Concat1/1
  Concat1/1 -> Slice/1

== system aurora_cpu_ch0_ver2_rtxsg/StatusPacker1/Subsystem/Subsystem2 ==
  In1 : Inport
  Concat1 : xbsIndex_r4/Concat  num_inputs=2  dbl_ovrd=off  block_type=concat
  Constant3 : xbsIndex_r4/Constant  const=0  gui_display_data_type=Fixed-point  arith_type=Unsigned  n_bits=32  bin_pt=0  preci_type=Single  exp_width=8  frac_width=24  explicit_period=on  period=opGetFPGAPeriod(bdroot)  equ=P=C  opselect=C  inp2=PCIN>>17  opr=+  inp1=P  carry=CIN  dbl_ovrd=off  block_type=constant
  Slice : xbsIndex_r4/Slice  nbits=32  boolean_output=off  mode=Lower Bit Location + Width  bit1=0  base1=MSB of Input  bit0=0  base0=LSB of Input  dbl_ovrd=off  block_type=slice
  Out1 : Outport
  wires:
  Concat1/1 -> Slice/1
  Constant3/1 -> Concat1/1
  Slice/1 -> Out1/1
  In1/1 -> Concat1/2

== system aurora_cpu_ch0_ver2_rtxsg/StatusPacker1/Subsystem/Subsystem3 ==
  In1 : Inport
  Concat1 : xbsIndex_r4/Concat  num_inputs=2  dbl_ovrd=off  block_type=concat
  Constant3 : xbsIndex_r4/Constant  const=0  gui_display_data_type=Fixed-point  arith_type=Unsigned  n_bits=32  bin_pt=0  preci_type=Single  exp_width=8  frac_width=24  explicit_period=on  period=opGetFPGAPeriod(bdroot)  equ=P=C  opselect=C  inp2=PCIN>>17  opr=+  inp1=P  carry=CIN  dbl_ovrd=off  block_type=constant
  Slice : xbsIndex_r4/Slice  nbits=32  boolean_output=off  mode=Lower Bit Location + Width  bit1=0  base1=MSB of Input  bit0=0  base0=LSB of Input  dbl_ovrd=off  block_type=slice
  Out1 : Outport
  wires:
  In1/1 -> Concat1/2
  Slice/1 -> Out1/1
  Constant3/1 -> Concat1/1
  Concat1/1 -> Slice/1

== system aurora_cpu_ch0_ver2_rtxsg/StatusPacker1/Subsystem/Subsystem4 ==
  In1 : Inport
  Concat1 : xbsIndex_r4/Concat  num_inputs=2  dbl_ovrd=off  block_type=concat
  Constant3 : xbsIndex_r4/Constant  const=0  gui_display_data_type=Fixed-point  arith_type=Unsigned  n_bits=32  bin_pt=0  preci_type=Single  exp_width=8  frac_width=24  explicit_period=on  period=opGetFPGAPeriod(bdroot)  equ=P=C  opselect=C  inp2=PCIN>>17  opr=+  inp1=P  carry=CIN  dbl_ovrd=off  block_type=constant
  Slice : xbsIndex_r4/Slice  nbits=32  boolean_output=off  mode=Lower Bit Location + Width  bit1=0  base1=MSB of Input  bit0=0  base0=LSB of Input  dbl_ovrd=off  block_type=slice
  Out1 : Outport
  wires:
  Concat1/1 -> Slice/1
  Constant3/1 -> Concat1/1
  Slice/1 -> Out1/1
  In1/1 -> Concat1/2

== system aurora_cpu_ch0_ver2_rtxsg/StatusPacker1/Subsystem/Subsystem5 ==
  In1 : Inport
  Concat1 : xbsIndex_r4/Concat  num_inputs=2  dbl_ovrd=off  block_type=concat
  Constant3 : xbsIndex_r4/Constant  const=0  gui_display_data_type=Fixed-point  arith_type=Unsigned  n_bits=32  bin_pt=0  preci_type=Single  exp_width=8  frac_width=24  explicit_period=on  period=opGetFPGAPeriod(bdroot)  equ=P=C  opselect=C  inp2=PCIN>>17  opr=+  inp1=P  carry=CIN  dbl_ovrd=off  block_type=constant
  Slice : xbsIndex_r4/Slice  nbits=32  boolean_output=off  mode=Lower Bit Location + Width  bit1=0  base1=MSB of Input  bit0=0  base0=LSB of Input  dbl_ovrd=off  block_type=slice
  Out1 : Outport
  wires:
  In1/1 -> Concat1/2
  Slice/1 -> Out1/1
  Constant3/1 -> Concat1/1
  Concat1/1 -> Slice/1

== system aurora_cpu_ch0_ver2_rtxsg/Synchronization/UserTstepPulse_Prediction/ModelRst ==
  Convert3 : xbsIndex_r4/Convert  gui_display_data_type=Boolean  arith_type=Boolean  n_bits=16  bin_pt=14  float_type=Single  exp_bits=8  fraction_bits=24  quantization=Truncate  overflow=Wrap  en=off  latency=0  pipeline=off  dbl_ovrd=off  block_type=convert
  Inverter1 : xbsIndex_r4/Inverter  en=off  latency=0  dbl_ovrd=off  block_type=inv
  Simulation State : rtxsg_common/Simulation State  TimerWidth=22
      settings: SourceProductName=RT-XSG
  Rst : Outport
  wires:
  Inverter1/1 -> Convert3/1
  Simulation State/3 -> Inverter1/1
  Convert3/1 -> Rst/1
